simulink model "Pacemaker"  (R2022a)
settings: Solver=FixedStepAuto  StartTime=0.0  StopTime=10.0  FixedStep=1e-3  RelTol=1e-3  EnableMultiTasking=on
undefined symbols (not defined in the file or in its folder): Pacemaker_Mode
libraries: simulink x1, frdmk64flib x1
settings Model: ExtModeTrigDuration=5  Creator=ivanl  LastModifiedBy=ivanl
settings SolverCC: AlgebraicLoopSolver=TrustRegion
settings OptimizationCC: EnhancedBackFolding=on  PassReuseOutputArgsAs=Individual arguments  ZeroExternalMemoryAtStartup=off  ZeroInternalMemoryAtStartup=off  MaxStackSize=64  OptimizeBlockOrder=speed  DifferentSizesBufferReuse=on  OptimizationCustomize=off  EfficientTunableParamExpr=on
settings DebuggingCC: ParameterTunabilityLossMsg=error  UnconnectedInputMsg=warning  UnconnectedOutputMsg=warning  UnconnectedLineMsg=warning  SFMachineParentedDataDiag=warning
settings HardwareCC: ProdBitPerPointer=32  ProdBitPerSizeT=32  ProdBitPerPtrDiffT=32  ProdLargestAtomicInteger=Long  ProdLargestAtomicFloat=Double  ProdWordSize=32  ProdHWDeviceType=ARM Compatible->ARM Cortex
settings SFSimCC: MATLABDynamicMemAlloc=off
settings RTWCC: SystemTargetFile=ert.tlc  HardwareBoard=NXP FRDM-K64F  TLCOptions="-aInlineSetEventsForThisBaseRateFcn=TLC_FALSE -aSuppressMultiTaskScheduler=TLC_FALSE  -aRateBasedStepFcn=0"  TemplateMakefile=ert_default_tmf  Toolchain=GNU Tools for ARM Embedded Processors
settings CodeAppCC: ForceParamTrailComments=on  IgnoreCustomStorageClasses=off  OperatorAnnotations=on  SimulinkDataObjDesc=on  SFDataObjDesc=on  InsertBlockDesc=on

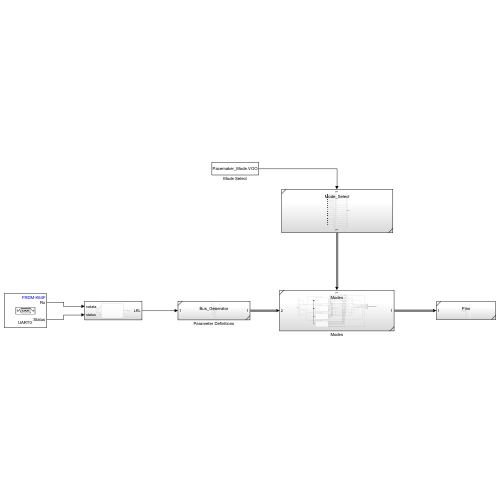
[thumbnail: Simulink's stored preview of the top-level diagram]
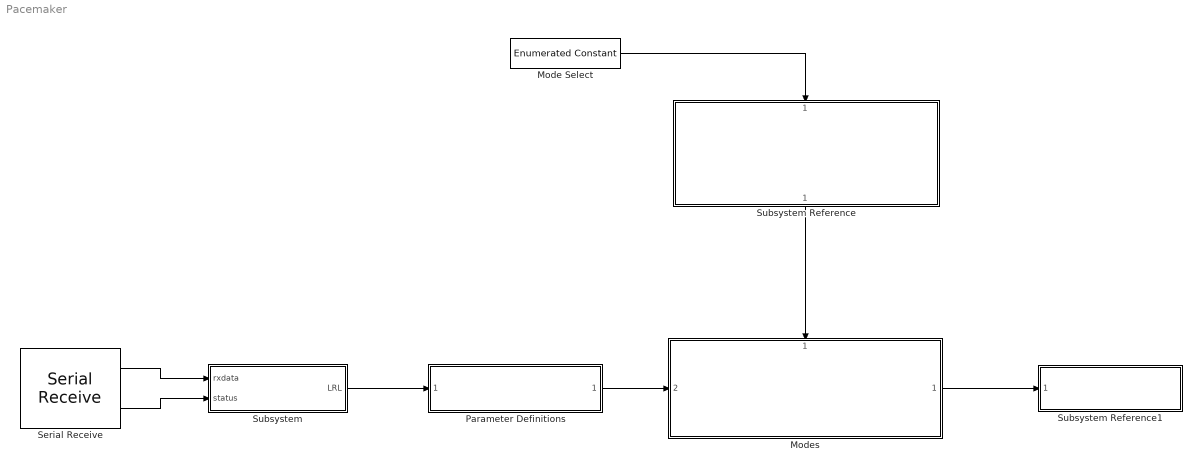
== system Pacemaker ==
  Mode Select : simulink/Sources/Enumerated Constant  OutDataTypeStr=Enum: Pacemaker_Mode  Value=Pacemaker_Mode.VOO  SampleTime=inf
  Modes : Subsystem  ReferencedSubsystem=Modes
      settings: PortSchema="{\"entries\":[{\"content\":{\"sides\":[{\"content\":{\"connectorIds\":[\"In2\"]},\"type\":\"ConnectorPlacement.EquallySpacedRectSide\",\"uuid\":\"23b6e2de-0d65-44c6-b999-78ff36285303\"},{\"content\":{\"connectorIds\":[\"Out1\"],\"side\":\"RIGHT\"},\"type\":\"ConnectorPlacement.EquallySpacedRectSide\",\"uuid\":\"6e379e72-2c3b-4826-965e-c3ade9111507\"},{\"content\":{\"connectorIds\":[\"In1\"],\"side\":\"TOP\"},\"type\":\"ConnectorPlacement.EquallySpacedRectSide\",\"uuid\":\"02099858-294b-4eb9-9c6c-4f00a8f85291\"}]},\"type\":\"ConnectorPlacement.EquallySpacedConnector\",\"uuid\":\"d9b74c95-6958-4d8f-a533-9e43d6dcc444\"}],\"packageUris\":[\"http://schema.mathworks.com/mf0/Connector/R2020b\"],\"version\":\"1.0\"}"
  Parameter Definitions : Subsystem  ReferencedSubsystem=Bus_Generator
  Serial Receive : frdmk64flib/Serial Receive  SCIModule=0  Baudrate=uint32(9600)  Parity=None  StopBits=1  HardwareFlowControl=None  ByteOrder=LittleEndian  DataType=uint8  DataLength=1  BlockingMode=off  OutputStatus=on  SampleTime=0.1
  Subsystem : Subsystem
  Subsystem Reference : Subsystem  ReferencedSubsystem=Mode_Select
      settings: PortSchema="{\"entries\":[{\"content\":{\"sides\":[{\"content\":{\"connectorIds\":[]},\"type\":\"ConnectorPlacement.EquallySpacedRectSide\",\"uuid\":\"5818db6d-40b9-4663-a28c-b99e994c8c04\"},{\"content\":{\"connectorIds\":[],\"side\":\"RIGHT\"},\"type\":\"ConnectorPlacement.EquallySpacedRectSide\",\"uuid\":\"617f5f9f-470b-42ea-b3a6-edd8f032ea28\"},{\"content\":{\"connectorIds\":[\"In1\"],\"side\":\"TOP\"},\"type\":\"ConnectorPlacement.EquallySpacedRectSide\",\"uuid\":\"87ea0b53-5d8d-433a-b8ed-41456f30d2be\"},{\"content\":{\"connectorIds\":[\"Out1\"],\"side\":\"BOTTOM\"},\"type\":\"ConnectorPlacement.EquallySpacedRectSide\",\"uuid\":\"0a78aeab-4e50-420e-8ed1-115a26d5575f\"}]},\"type\":\"ConnectorPlacement.EquallySpacedConnector\",\"uuid\":\"77f4e980-0bdf-45c1-b4ca-33966fa0c89e\"}],\"packageUris\":[\"http://schema.mathworks.com/mf0/Connector/R2020b\"],\"version\":\"1.0\"}"
  Subsystem Reference1 : Subsystem  ReferencedSubsystem=Pins
  wires:
  Mode Select/1 -> Subsystem Reference/1
  Modes/1 -> Subsystem Reference1/1
  Parameter Definitions/1 -> Modes/2
  Subsystem Reference/1 -> Modes/1
  Serial Receive/1 -> Subsystem/1(rxdata)
  Serial Receive/2 -> Subsystem/2(status)
  Subsystem/1(LRL) -> Parameter Definitions/1

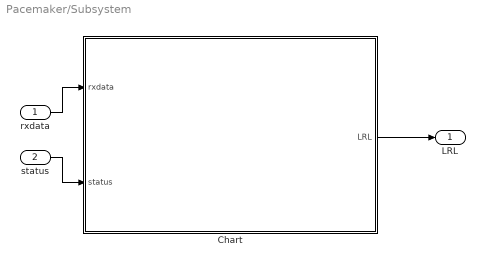
== system Pacemaker/Subsystem ==
  rxdata : Inport
  status : Inport  Port=2
  Chart : Stateflow chart  TreatAsAtomicUnit=on
  LRL : Outport
  wires:
  rxdata/1 -> Chart/1(rxdata)
  status/1 -> Chart/2(status)
  Chart/1(LRL) -> LRL/1

== stateflow chart Pacemaker/Subsystem/Chart ==
  state SET_PARAMS
    entry:
    LRL = rxdata(1:2);
  state DEFAULT
    entry:
    LRL = 60;
    URL = 60;
  state STANDBY
  (default) -> DEFAULT
  SET_PARAMS -> STANDBY
  DEFAULT -> STANDBY
  STANDBY -> (junction 8) : [status == 0]
  (junction 8) -> SET_PARAMS
  data: rxdata input uint8; status input uint8; LRL output uint8; URL local uint8
